simulink model "Lab3_Parte2"  (R2017a)
settings: Solver=VariableStepAuto  StartTime=0.0  StopTime=10.0  RelTol=1e-3
libraries: simulink x3, simulink_extras x1
settings Model: Creator=jaraya  LastModifiedBy=Diego
settings DataIOCC: LimitDataPoints=on  SaveOutput=off  SaveTime=off
settings OptimizationCC: BlockReduction=off  BooleanDataType=off  LifeSpan=inf
settings DebuggingCC: SaveWithParameterizedLinksMsg=none  UnderspecifiedInitializationDetection=Classic  MergeDetectMultiDrivingBlocksExec=none  SignalResolutionControl=TryResolveAllWithWarning  AllowSymbolicDim=off  SFUnexpectedBacktrackingDiag=warning  SFNoUnconditionalDefaultTransitionDiag=warning  SFExecutionAtInitializationDiag=none
settings HardwareCC: TargetUnknown=on
settings GRTTargetCC: TargetLangStandard=C89/C90 (ANSI)  GeneratePreprocessorConditionals=Disable all

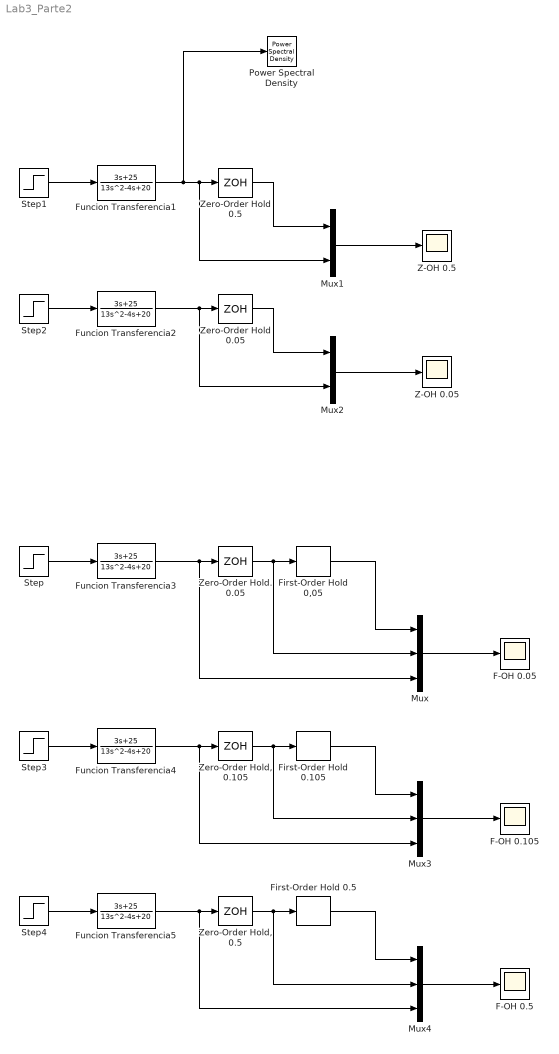
== system Lab3_Parte2 ==
  F-OH 0.05 : Scope
  F-OH 0.105 : Scope
  F-OH 0.5 : Scope
  First-Order Hold 0,05 : simulink/Discrete/First-Order Hold  DisableCoverage=on  Ts=0.05
      settings: SourceProductName=Simulink  SourceProductBaseCode=SL
  First-Order Hold 0.105 : simulink/Discrete/First-Order Hold  DisableCoverage=on  Ts=0.105
      settings: SourceProductName=Simulink  SourceProductBaseCode=SL
  First-Order Hold 0.5 : simulink/Discrete/First-Order Hold  DisableCoverage=on  Ts=0.5
      settings: SourceProductName=Simulink  SourceProductBaseCode=SL
  Funcion Transferencia{1..5} (5 alike) : TransferFcn  Numerator=[3 25]  Denominator=[13 -4 20]
  Mux : Mux  Inputs=3
  Mux1 : Mux  Inputs=2
  Mux2 : Mux  Inputs=2
  Mux3 : Mux  Inputs=3
  Mux4 : Mux  Inputs=3
  Power Spectral Density : simulink_extras/Additional Sinks/Power Spectral Density  npts=128  fftpts=512  HowOften=64  sampleT=0.1
      settings: SourceProductName=Simulink  SourceProductBaseCode=SL
  Step{,1..4} (5 alike) : Step  SampleTime=0
  Z-OH 0.05 : Scope
  Z-OH 0.5 : Scope
  Zero-Order Hold 0.05 : ZeroOrderHold  SampleTime=0.05
  Zero-Order Hold 0.5 : ZeroOrderHold  SampleTime=0.5
  "Zero-Order Hold, 0.105" : ZeroOrderHold  SampleTime=0.105
  "Zero-Order Hold, 0.5" : ZeroOrderHold  SampleTime=0.5
  Zero-Order Hold. 0.05 : ZeroOrderHold  SampleTime=0.05
  wires:
  Step/1 -> Funcion Transferencia3/1
  Funcion Transferencia3/1 -> Mux/3, Zero-Order Hold. 0.05/1
  Zero-Order Hold. 0.05/1 -> Mux/2, First-Order Hold 0,05/1
  First-Order Hold 0,05/1 -> Mux/1
  Mux/1 -> F-OH 0.05/1
  Zero-Order Hold 0.5/1 -> Mux1/1
  Mux1/1 -> Z-OH 0.5/1
  Funcion Transferencia1/1 -> Power Spectral Density/1, Mux1/2, Zero-Order Hold 0.5/1
  Step1/1 -> Funcion Transferencia1/1
  Zero-Order Hold 0.05/1 -> Mux2/1
  Mux2/1 -> Z-OH 0.05/1
  Funcion Transferencia2/1 -> Mux2/2, Zero-Order Hold 0.05/1
  Step2/1 -> Funcion Transferencia2/1
  "Zero-Order Hold, 0.105"/1 -> Mux3/2, First-Order Hold 0.105/1
  Mux3/1 -> F-OH 0.105/1
  Funcion Transferencia4/1 -> Mux3/3, "Zero-Order Hold, 0.105"/1
  First-Order Hold 0.105/1 -> Mux3/1
  Step3/1 -> Funcion Transferencia4/1
  Mux4/1 -> F-OH 0.5/1
  "Zero-Order Hold, 0.5"/1 -> Mux4/2, First-Order Hold 0.5/1
  Step4/1 -> Funcion Transferencia5/1
  First-Order Hold 0.5/1 -> Mux4/1
  Funcion Transferencia5/1 -> Mux4/3, "Zero-Order Hold, 0.5"/1
